simulink model "Model_Simscape_V3"  (R2023a)
settings: Solver=VariableStepAuto  StartTime=0.0  StopTime=10.0  RelTol=1e-3
model workspace (MAT data in the model file):
  Air_density = 1.29
  Body_Temperature = 37
  CtrlData_Max = 100
  CtrlData_Min = 0
  Detpress_to_Vavle.detpress = [1.45 1.55 1.6 1.65 1.7 1.75 1.8 1.85 1.9 1.95 2 2.05 5 7 26 42 60 78 99 112]
  Detpress_to_Vavle.vavle = [0.999 0.94 0.89 0.84 0.78 0.73 0.68 0.63 0.57 0.52 0.47 0.42 0.36 0.31 0.25 0.21 0.15 0.1 0.05 0]
  E_respriatory = 10
  ExpValve.opening_vector = [0 0.052 0.105 0.157 0.21 0.263 0.315 0.368 0.421 0.473 0.526 0.578 0.631 0.684 0.736 0.789 0.842 0.894 0.947 1]
  ExpValve.Cv_vector = [0.0001 0.81 1.114 1.723 3.218 3.547 4.603 5.2063 6.069 6.57 6.974 7.226 7.563 7.856 7.997 8.565 8.84 9.267 9.621 10.487]
  ExpValve.threshold = 0.0011
  ExpValve.zerovalue = 0
  ExpValve.Cross_Area = 0.000314159265359
  ExpValve.fullValue = 1
  FRC = 2
  Fan.shaftspeed = [14400 15600 16800 18000 19200 20400 21600 22800 24000 25200 26400 27600 28800 30000 31200 32400 33600 34800 36000 37200 38400 39600 40800 42000 43200 44400 45600 46800 48000]
  Fan.presstable = [0; 1; 2; 3; 4; 5; 6; 7; 8]
  Fan.flowvector = [97.5714285714 106 114 122 128.666666667 137 147.5 160.272727273 169.5 178.424242424 186.909090909 195.25 ... (261 elements, 29x9)]
  Fan.efficiency = [0.45  0.45  NaN  NaN  NaN  NaN  NaN  NaN  NaN; 0.45  0.45  NaN  NaN  NaN  NaN  NaN  NaN  NaN; 0.45  0.45  NaN  NaN  NaN  NaN  NaN  NaN  NaN; 0.45  0.45  NaN  NaN  NaN  NaN  NaN  NaN  NaN; 0.45  0.45  NaN  NaN  NaN  NaN  NaN  NaN  NaN; 0.45  0.45  NaN  NaN  NaN  NaN  NaN  NaN  NaN; 0.45  0.45  0.45  NaN  NaN  NaN  NaN  NaN  NaN; 0.45  0.45  0.45  NaN  NaN  NaN  NaN  NaN  NaN; 0.45  0.45  0.45  0.45  NaN  NaN  NaN  NaN  NaN; 0.45  0.45  0.45  0.45  NaN  NaN  NaN  NaN  NaN; 0.45  0.45  0.45  0.45  NaN  NaN  NaN  NaN  NaN; 0.45  0.45  0.45  0.45  NaN  NaN  NaN  NaN  NaN; 0.45  0.45  0.45  0.45  NaN  NaN  NaN  NaN  NaN; 0.45  0.45  0.45  0.45  0.45  NaN  NaN  NaN  NaN; 0.45  0.45  0.45  0.45  0.45  NaN  NaN  NaN  NaN; 0.45  0.45  0.45  0.45  0.45  NaN  NaN  NaN  NaN; 0.45  0.45  0.45  0.45  0.45  0.45  NaN  NaN  NaN; 0.45  0.45  0.45  0.45  0.45  0.45  NaN  NaN  NaN; 0.45  0.45  0.45  0.45  0.45  0.45  0.45  NaN  NaN; 0.45  0.45  0.45  0.45  0.45  0.45  0.45  NaN  NaN; 0.45  0.45  0.45  0.45  0.45  0.45  0.45  NaN  NaN; 0.45  0.45  0.45  0.45  0.45  0.45  0.45  NaN  NaN; 0.45  0.45  0.45  0.45  0.45  0.45  0.45  0.45  NaN; 0.45  0.45  0.45  0.45  0.45  0.45  0.45  0.45  NaN; 0.45  0.45  0.45  0.45  0.45  0.45  0.45  0.45  NaN; 0.45  0.45  0.45  0.45  0.45  0.45  0.45  0.45  0.45; 0.45  0.45  0.45  0.45  0.45  0.45  0.45  0.45  0.45; 0.45  0.45  0.45  0.45  0.45  0.45  0.45  0.45  0.45; 0.45  0.45  0.45  0.45  0.45  0.45  0.45  0.45  0.45]
  Fan.Inlerarea_A = 0.000314159265359
  Fan.Inlerarea_B = 0.000314159265359
  FanHousing.resistance = 1
  FanHousing.pressure_drop = 1
  FanHousing.flow_rate = 1
  FanHousing.Crosss_Area = 0.000314159265359
  FanHousing.Chamber_volume = 0.0001
  FanHousing.A_area = 0.000314159265359
  FanHousing.B_area = 0.000314159265359
  FanHousing.C_area = 0.000314159265359
  Flow_Resistance_1.resistance = 0.1
  Flow_Resistance_1.pressure_drop = 0.1
  Flow_Resistance_1.flow_rate = 1
  Flow_Resistance_1.Crosss_Area = 0.000314159265359
  Flow_Resistance_2.resistance = 0.1
  Flow_Resistance_2.pressure_drop = 0.1
  Flow_Resistance_2.flow_rate = 1
  Flow_Resistance_2.Crosss_Area = 0.000314159265359
  Hard_Stop.Lower_bound = -1e-06
  InspValve.opening_vector = [0 0.052 0.105 0.157 0.21 0.263 0.315 0.368 0.421 0.473 0.526 0.578 0.631 0.684 0.736 0.789 0.842 0.894 0.947 1]
  InspValve.Cv_vector = [0.0001 0.81 1.114 1.723 3.218 3.547 4.603 5.2063 6.069 6.57 6.974 7.226 7.563 7.856 7.997 8.565 8.84 9.267 9.621 10.487]
  InspValve.threshold = 0.0011
  InspValve.zerovalue = 0
  InspValve.Cross_Area = 0.000314159265359
  L_to_m3 = 0.001
  Mask.Chamber_volume = 0.0002
  Mask.A_area = 0.000314159265359
  Mask.B_area = 0.000314159265359
  Mask.C_area = 0.000314159265359
  OxyValve.Cv_vector = [0.0002693 0.0031 0.0081 0.0128 0.0184 0.0251 0.0321 0.039 0.046 0.0529 0.0604 0.0686 0.0742 0.082 0.0861 0.0918 0.0975 0.1032 0.1129 0.1156 0.1165]
  OxyValve.opening_vector = [0.5078 0.5334 0.559 0.5846 0.6102 0.6358 0.6614 0.687 0.7127 0.7383 0.7639 0.7895 0.8151 0.8407 0.8663 0.8919 0.9175 0.9431 0.9688 0.9944 1]
  OxyValve.Cross_Area = 0.000314159265359
  OxyValve.Pressure_Source = 500000
  OxygenSensor.Air_oxygen_concentration = 0.209
  OxygenSensor.K = 0.791
  Pa_to_cmH2O = 0.0101974428892
  Percent_to_Unit = 0.01
  Pipe_1.r = 0.01
  Pipe_1.longlength = 0.1
  Pipe_1.area = 0.000314159265359
  Pipe_1.diameter = 0.02
  Pipe_2.r = 0.01
  Pipe_2.longlength = 0.1
  Pipe_2.area = 0.000314159265359
  Pipe_2.diameter = 0.02
  Pipe_3.r = 0.01
  Pipe_3.longlength = 0.1
  Pipe_3.area = 0.000314159265359
  Pipe_3.diameter = 0.02
  R_respiratory = 2
  Reservoir.Cross_area = 0.000314159265359
  Trachea.Pipe_length = 0.15
  Trachea.area = 0.000314159265359
  Trachea.Hydraulic_diameter = 0.02
  Volume_Max = 0.9
  cmH2O_to_Pa = 98.0638
  cmH2O_to_kPa = 0.0981
  lung.Interface_area = 1
  lung.Dead_volume = 1e-06
  lung.Cross_area = 0.000314159265359
  percentage_to_rpm = 600
values from neighbouring files (symbols this model uses):
  MIN_TO_S = 60.0    [MVEPP_DataDict.sldd]
  TO_HUNDRED = 0.01    [MVEPP_DataDict.sldd]
  TO_MILLI = 1000.0    [MVEPP_DataDict.sldd]
libraries: fl_lib x83, nesl_utility x17, SimscapeFluids_lib x4, aerolibatmos2 x1
(part 1 of 4)
settings Model: DataDictionary=MVEPP_DataDict.sldd  Creator=xuluyu  LastModifiedBy=yinjilai
settings SolverCC: DaesscMode=Fast
settings OptimizationCC: UseDivisionForNetSlopeComputation=on
settings SimscapeCC: SimscapeLogLimitData=off

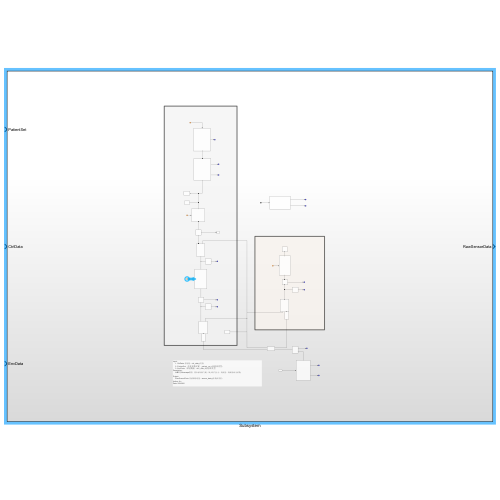
[thumbnail: Simulink's stored preview of the top-level diagram]
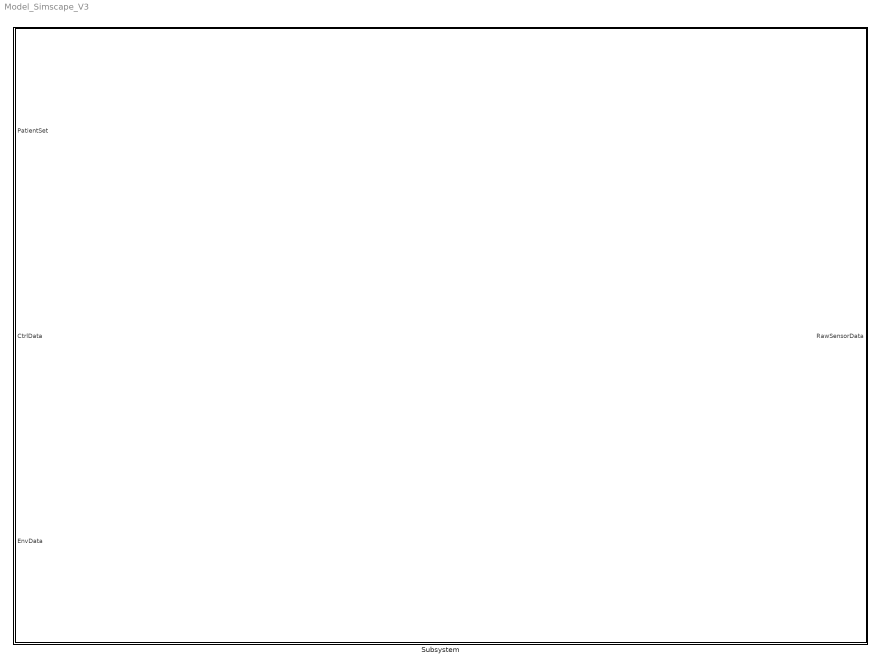
== system Model_Simscape_V3 ==
  Subsystem : Subsystem
